simulink model "threeDiskOscillatorRig_noFric"  (R2020a)
settings: Solver=VariableStepAuto  StartTime=0.0  StopTime=10  RelTol=1e-8
values from neighbouring files (symbols this model uses):
  b_1 = mean(ECP_values([6 7]))    [MandatoryAssignmentB_Loopsyn.m]    (also in MandatoryAssignmentB_Q13.m; MandatoryAssignmentB_Q9.m; threeDiskOscillator_9.m)
  b_2 = mean(ECP_values([8 9]))    [MandatoryAssignmentB_Loopsyn.m]    (also in MandatoryAssignmentB_Q13.m; MandatoryAssignmentB_Q9.m; threeDiskOscillator_9.m)
  b_3 = mean(ECP_values([10 11]))    [MandatoryAssignmentB_Loopsyn.m]    (also in MandatoryAssignmentB_Q13.m; MandatoryAssignmentB_Q9.m; threeDiskOscillator_9.m)
  J_1 = 0.0325    [MandatoryAssignmentB_Loopsyn.m]    (also in MandatoryAssignmentB_Q13.m; MandatoryAssignmentB_Q15.m = ECP_values(1); MandatoryAssignmentB_Q9.m = ECP_values(1); threeDiskOscillator_9.m = ECP_values(1))
  J_2 = ECP_values(2)    [MandatoryAssignmentB_Loopsyn.m]    (also in MandatoryAssignmentB_Q13.m; MandatoryAssignmentB_Q9.m; threeDiskOscillator_9.m)
  J_3 = ECP_values(3)    [MandatoryAssignmentB_Loopsyn.m]    (also in MandatoryAssignmentB_Q13.m; MandatoryAssignmentB_Q9.m; threeDiskOscillator_9.m)
  k_1 = ECP_values(4)    [MandatoryAssignmentB_Loopsyn.m]    (also in MandatoryAssignmentB_Q13.m; MandatoryAssignmentB_Q9.m; threeDiskOscillator_9.m)
  k_2 = ECP_values(5)    [MandatoryAssignmentB_Loopsyn.m]    (also in MandatoryAssignmentB_Q13.m; MandatoryAssignmentB_Q9.m; threeDiskOscillator_9.m)
  T_s = 0.004    [MandatoryAssignmentB_Q13.m]    (also in MandatoryAssignmentB_Q14.m = 0.0004; MandatoryAssignmentB_Q14_RP.m = 0.0004; MandatoryAssignmentB_Q14_messy.m = 0.0004; MandatoryAssignmentB_Q9.m = 0.0004)
  x_0 = [0;0;0;0;0;0]    [MandatoryAssignmentB_Q14.m]    (also in MandatoryAssignmentB_Q14_RP.m; MandatoryAssignmentB_Q14_messy.m; MandatoryAssignmentB_Q9.m; threeDiskOscillator_9.m)
undefined symbols (not defined in the file or in its folder): denK, denW1, denW2, numK, numW1, numW2
libraries: simulink x1
settings Model: Creator=dimpa  LastModifiedBy=Administrator
settings DataIOCC: ReturnWorkspaceOutputs=off
settings DebuggingCC: ArithmeticOperatorsInVariantConditions=warning
settings SFSimCC: SimUseLocalCustomCode=off  CustomCodeUndefinedFunction=UseInterfaceOnly
settings RTWCC: RTWUseLocalCustomCode=off

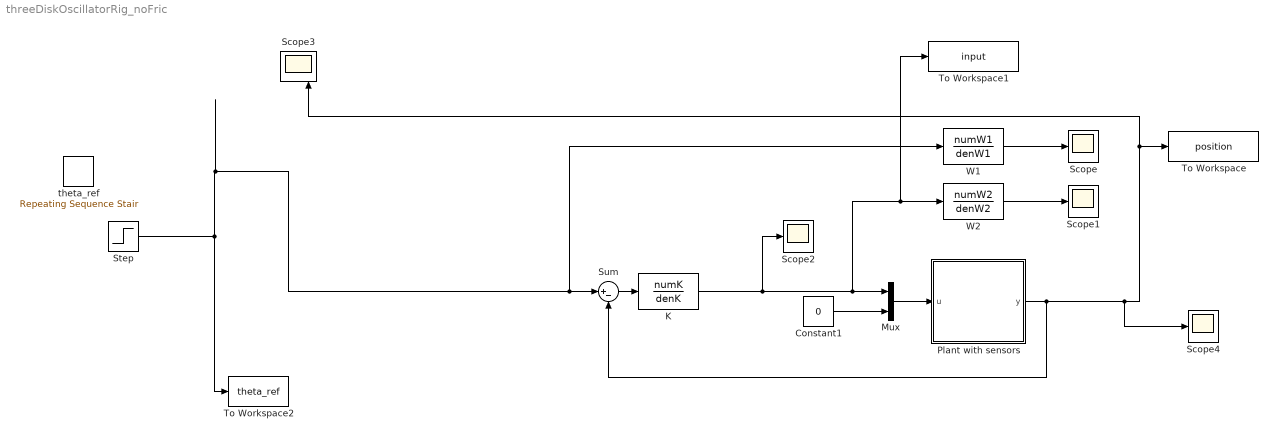
== system threeDiskOscillatorRig_noFric ==
  Constant1 : Constant  Value=0
  K : TransferFcn  Numerator=numK  Denominator=denK
  Mux : Mux  Inputs=2
  Plant with sensors : Subsystem
  Scope{,1..2,4} (4 alike) : Scope
  Scope3 : Scope  NumInputPorts=2
  Step : Step  Time=0  SampleTime=0
  Sum : Sum  Inputs=|+-
  To Workspace : ToWorkspace  VariableName=position  SaveFormat=Timeseries  SampleTime=-1
  To Workspace1 : ToWorkspace  VariableName=input  SaveFormat=Timeseries  SampleTime=-1
  To Workspace2 : ToWorkspace  VariableName=theta_ref  SaveFormat=Timeseries  SampleTime=T_s
  W1 : TransferFcn  Numerator=numW1  Denominator=denW1
  W2 : TransferFcn  Numerator=numW2  Denominator=denW2
  theta_ref : simulink/Sources/Repeating Sequence Stair  OutValues=[0 1.57 0]  tsamp=5  OutMin=[]  OutMax=[]  OutDataTypeStr=double  OutputDataTypeScalingMode=double  OutDataType=fixdt(0,8)  ConRadixGroup=Best Precision: Vector-wise  OutScaling=2^-12
  wires:
  Plant with sensors/1(y) -> Scope4/1, To Workspace/1, Scope3/2, Sum/2
  Sum/1 -> K/1
  Constant1/1 -> Mux/2
  Mux/1 -> Plant with sensors/1(u)
  W1/1 -> Scope/1
  W2/1 -> Scope1/1
  Step/1 -> W1/1, Sum/1, To Workspace2/1
  K/1 -> Scope2/1, To Workspace1/1, W2/1, Mux/1

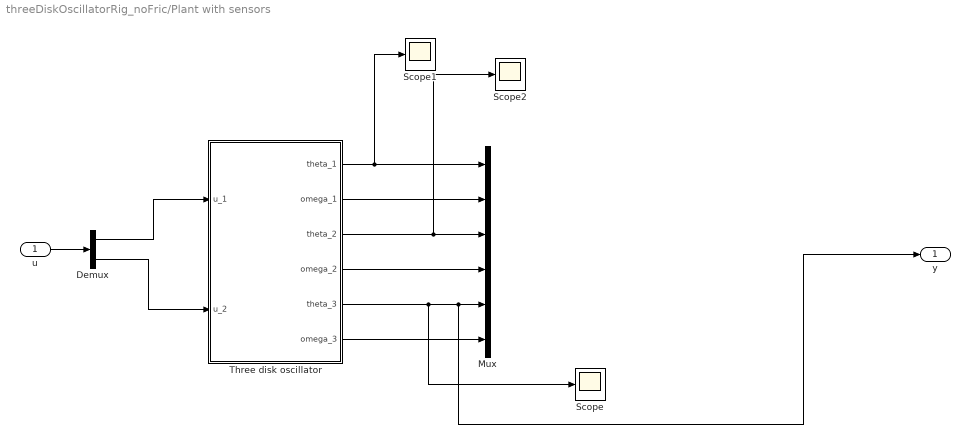
== system threeDiskOscillatorRig_noFric/Plant with sensors ==
  u : Inport
  Demux : Demux  Outputs=2
  Mux : Mux  Inputs=6
  Scope : Scope
  Scope1 : Scope
  Scope2 : Scope
  Three disk oscillator : Subsystem
  y : Outport  VectorParamsAs1DForOutWhenUnconnected=off
  wires:
  u/1 -> Demux/1
  Three disk oscillator/2(omega_1) -> Mux/2
  Three disk oscillator/1(theta_1) -> Scope1/1, Mux/1
  Three disk oscillator/4(omega_2) -> Mux/4
  Three disk oscillator/3(theta_2) -> Scope2/1, Mux/3
  Three disk oscillator/6(omega_3) -> Mux/6
  Demux/2 -> Three disk oscillator/2(u_2)
  Demux/1 -> Three disk oscillator/1(u_1)
  Three disk oscillator/5(theta_3) -> Scope/1, y/1, Mux/5

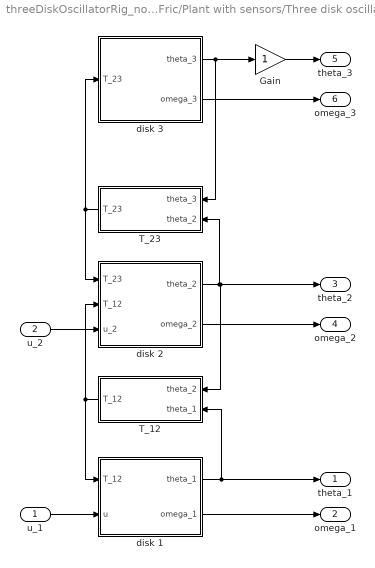
== system threeDiskOscillatorRig_noFric/Plant with sensors/Three disk oscillator ==
  u_1 : Inport
  u_2 : Inport  Port=2
  Gain : Gain
  T_12 : Subsystem
  T_23 : Subsystem
  disk 1 : Subsystem
  disk 2 : Subsystem
  disk 3 : Subsystem
  theta_1 : Outport  VectorParamsAs1DForOutWhenUnconnected=off
  omega_1 : Outport  Port=2  VectorParamsAs1DForOutWhenUnconnected=off
  theta_2 : Outport  Port=3  VectorParamsAs1DForOutWhenUnconnected=off
  omega_2 : Outport  Port=4  VectorParamsAs1DForOutWhenUnconnected=off
  theta_3 : Outport  Port=5  VectorParamsAs1DForOutWhenUnconnected=off
  omega_3 : Outport  Port=6  VectorParamsAs1DForOutWhenUnconnected=off
  wires:
  T_23/1(T_23) -> disk 2/1(T_23), disk 3/1(T_23)
  disk 1/1(theta_1) -> T_12/2(theta_1), theta_1/1
  disk 2/1(theta_2) -> T_23/2(theta_2), theta_2/1, T_12/1(theta_2)
  T_12/1(T_12) -> disk 1/1(T_12), disk 2/2(T_12)
  disk 3/2(omega_3) -> omega_3/1
  disk 1/2(omega_1) -> omega_1/1
  disk 2/2(omega_2) -> omega_2/1
  u_1/1 -> disk 1/2(u)
  disk 3/1(theta_3) -> Gain/1, T_23/1(theta_3)
  Gain/1 -> theta_3/1
  u_2/1 -> disk 2/3(u_2)

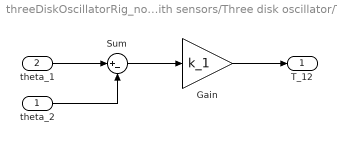
== system threeDiskOscillatorRig_noFric/Plant with sensors/Three disk oscillator/T_12 ==
  theta_2 : Inport
  theta_1 : Inport  Port=2
  Gain : Gain  Gain=k_1
  Sum : Sum  Inputs=|+-
  T_12 : Outport  VectorParamsAs1DForOutWhenUnconnected=off
  wires:
  theta_2/1 -> Sum/2
  theta_1/1 -> Sum/1
  Sum/1 -> Gain/1
  Gain/1 -> T_12/1

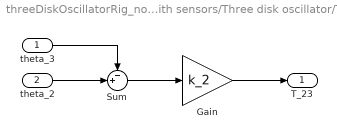
== system threeDiskOscillatorRig_noFric/Plant with sensors/Three disk oscillator/T_23 ==
  theta_3 : Inport
  theta_2 : Inport  Port=2
  Gain : Gain  Gain=k_2
  Sum : Sum  Inputs=-+|
  T_23 : Outport  VectorParamsAs1DForOutWhenUnconnected=off
  wires:
  Gain/1 -> T_23/1
  Sum/1 -> Gain/1
  theta_3/1 -> Sum/1
  theta_2/1 -> Sum/2

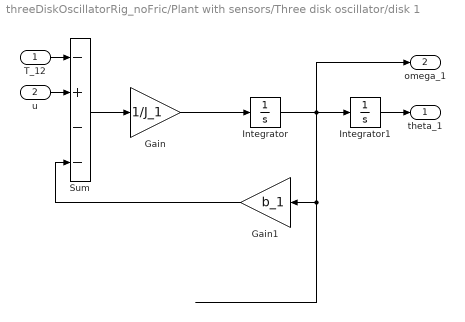
== system threeDiskOscillatorRig_noFric/Plant with sensors/Three disk oscillator/disk 1 ==
  T_12 : Inport
  u : Inport  Port=2
  Gain : Gain  Gain=1/J_1
  Gain1 : Gain  Gain=b_1
  Integrator : Integrator  InitialCondition=x_0(2)
  Integrator1 : Integrator  InitialCondition=x_0(1)
  Sum : Sum  Inputs=-+--
  theta_1 : Outport  VectorParamsAs1DForOutWhenUnconnected=off
  omega_1 : Outport  Port=2  VectorParamsAs1DForOutWhenUnconnected=off
  wires:
  Sum/1 -> Gain/1
  Integrator/1 -> Integrator1/1, omega_1/1, Gain1/1
  Gain1/1 -> Sum/4
  Integrator1/1 -> theta_1/1
  T_12/1 -> Sum/1
  u/1 -> Sum/2
  Gain/1 -> Integrator/1
  ? -> Sum/3

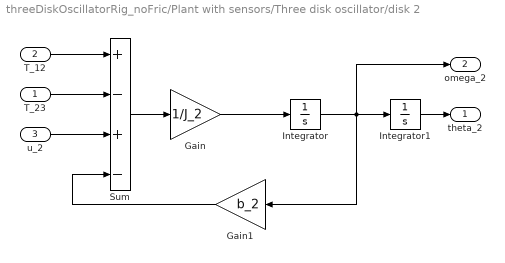
== system threeDiskOscillatorRig_noFric/Plant with sensors/Three disk oscillator/disk 2 ==
  T_23 : Inport
  T_12 : Inport  Port=2
  u_2 : Inport  Port=3
  Gain : Gain  Gain=1/J_2
  Gain1 : Gain  Gain=b_2
  Integrator : Integrator  InitialCondition=x_0(4)
  Integrator1 : Integrator  InitialCondition=x_0(3)
  Sum : Sum  Inputs=+-+-
  theta_2 : Outport  VectorParamsAs1DForOutWhenUnconnected=off
  omega_2 : Outport  Port=2  VectorParamsAs1DForOutWhenUnconnected=off
  wires:
  T_23/1 -> Sum/2
  T_12/1 -> Sum/1
  Integrator1/1 -> theta_2/1
  Gain1/1 -> Sum/4
  Gain/1 -> Integrator/1
  Integrator/1 -> Integrator1/1, Gain1/1, omega_2/1
  Sum/1 -> Gain/1
  u_2/1 -> Sum/3

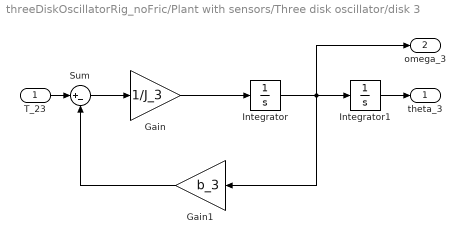
== system threeDiskOscillatorRig_noFric/Plant with sensors/Three disk oscillator/disk 3 ==
  T_23 : Inport
  Gain : Gain  Gain=1/J_3
  Gain1 : Gain  Gain=b_3
  Integrator : Integrator  InitialCondition=x_0(6)
  Integrator1 : Integrator  InitialCondition=x_0(5)
  Sum : Sum  Inputs=|+-
  theta_3 : Outport  VectorParamsAs1DForOutWhenUnconnected=off
  omega_3 : Outport  Port=2  VectorParamsAs1DForOutWhenUnconnected=off
  wires:
  Sum/1 -> Gain/1
  Integrator/1 -> Integrator1/1, omega_3/1, Gain1/1
  Gain/1 -> Integrator/1
  Gain1/1 -> Sum/2
  Integrator1/1 -> theta_3/1
  T_23/1 -> Sum/1
